simulink model "flatnessGen"  (R2016a)
settings: Solver=VariableStepAuto  StartTime=0.0  StopTime=30.0  RelTol=1e-3
settings Model: Creator=mgreiff  LastModifiedBy=mgreiff

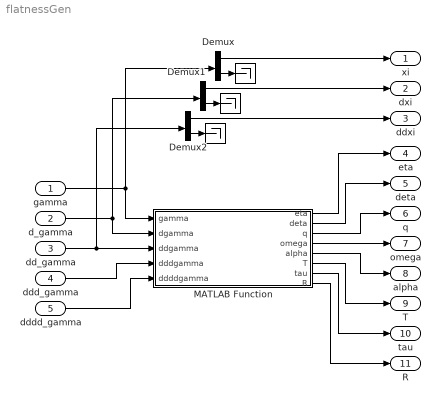
== system flatnessGen ==
  gamma : Inport  PortDimensions=4
  d_gamma : Inport  Port=2  PortDimensions=4
  dd_gamma : Inport  Port=3  PortDimensions=4
  ddd_gamma : Inport  Port=4  PortDimensions=4
  dddd_gamma : Inport  Port=5  PortDimensions=4
  " " : Terminator
  "   " : Terminator
  "    " : Terminator
  Demux : Demux  Outputs=[3,1]
  Demux1 : Demux  Outputs=[3,1]
  Demux2 : Demux  Outputs=[3,1]
  MATLAB Function : MATLAB Function  TreatAsAtomicUnit=on
  xi : Outport
  dxi : Outport  Port=2
  ddxi : Outport  Port=3
  eta : Outport  Port=4
  deta : Outport  Port=5
  q : Outport  Port=6
  omega : Outport  Port=7
  alpha : Outport  Port=8
  T : Outport  Port=9
  tau : Outport  Port=10
  R : Outport  Port=11
  wires:
  MATLAB Function/1(eta) -> eta/1
  MATLAB Function/2(deta) -> deta/1
  MATLAB Function/3(q) -> q/1
  MATLAB Function/4(omega) -> omega/1
  MATLAB Function/6(T) -> T/1
  MATLAB Function/7(tau) -> tau/1
  MATLAB Function/5(alpha) -> alpha/1
  gamma/1 -> Demux/1, MATLAB Function/1(gamma)
  dd_gamma/1 -> Demux2/1, MATLAB Function/3(ddgamma)
  d_gamma/1 -> Demux1/1, MATLAB Function/2(dgamma)
  dddd_gamma/1 -> MATLAB Function/5(ddddgamma)
  ddd_gamma/1 -> MATLAB Function/4(dddgamma)
  MATLAB Function/8(R) -> R/1
  Demux/2 -> " "/1
  Demux1/2 -> "   "/1
  Demux1/1 -> dxi/1
  Demux/1 -> xi/1
  Demux2/2 -> "    "/1
  Demux2/1 -> ddxi/1

== matlab function flatnessGen/MATLAB Function ==
  data: gamma input; eta output; dgamma input; ddgamma input; dddgamma input; ddddgamma input; deta output; q output; omega output; alpha output; T output; tau output; R output
function [eta, deta, q, omega, alpha, T, tau, R] = flatness(gamma, dgamma, ddgamma, dddgamma, ddddgamma)
%#codegen

% Thrust
g = 9.81;
m = 0.027;
I = diag([0.1660e-4; 0.1660e-4; 0.2930e-4]);
a = ddgamma(1:3);
atilde = a + [0;0;g];
T = m*norm(atilde);

% ~~~ Angles ~~~
psi = gamma(4);
zb = atilde./norm(atilde);
yc = [cos(psi+pi/2); sin(psi+pi/2); 0];
xb = cross(yc, zb)./norm(cross(yc, zb));
yb = cross(zb, xb);
R = [xb, yb, zb];

theta = -asin(R(3,1));
phi = atan2(R(3,2)/cos(theta), R(3,3)/cos(theta));

qsq = 0.25.*[ 1, 1, 1, 1; 1,-1,-1, 1; -1, 1,-1, 1; -1,-1, 1, 1] * [diag(R); 1];
q = sqrt(abs(qsq));
q(2) = q(2)* sign(R(3,2) - R(2,3));
q(3) = q(3)* sign(R(1,3) - R(3,1));
q(4) = q(4)* sign(R(2,1) - R(1,2));

eta = [phi; theta; psi];

% ~~~ Angular speeds ~~~
zw = [0;0;1];
dpsi = dgamma(4);
da = dddgamma(1:3);
pw = (m/T).*(da - (zb'*da).*zb);
A = [xb, yc, zw]\R;
omegax = -pw'*yb;
omegay = pw'*xb;
omegaz = (dpsi - A(3,1)*omegax - A(3,2)*omegay)/A(3,3);
omega = [omegax;omegay;omegaz];

dphi = A(1,:)*omega;
dtheta = A(2,:)*omega;
deta = [dphi; dtheta; dpsi];

% ~~~ Angular accelerations ~~~
da = dddgamma(1:3);
dda = ddddgamma(1:3);
ddpsi = ddgamma(4);

v = m.*dda - cross(omega, cross(omega, T*zb));
pa = (1/T)*(v - (zb'*v).*zb - 2.*cross(omega, m.*(zb'*da).*zb));
alphax = -pa'*yb;
alphay = pa'*xb;

omegacross = [0, -omegaz, omegay; omegaz, 0, -omegax; -omegay, omegax, 0];
omegac = [0;0;omegaz];
b = [xb, yc, zw]\((omegacross*R)*omega - cross(omega, dphi*xb) - cross(omegac, dtheta*yc));
alphaz = (ddpsi - b(3) - A(3,1)*alphax - A(3,2)*alphay)/A(3,3);
alpha = [alphax; alphay; alphaz];

% ~~~ Torques ~~~
tau = I*alpha + cross(omega, I*omega);
